simulink model "Expriment_All2"  (R2014a)
settings: Solver=FixedStepDiscrete  SolverMode=SingleTasking  StartTime=0.0  StopTime=inf  FixedStep=0.01  RelTol=1e-3
PostLoadFcn:
  | h_RPStest = RPStest;
model workspace (MAT data in the model file):
  gtest = 0
undefined symbols (not defined in the file or in its folder): avert, avert_freq_factor, avert_gaze_dirs_chance, avert_gaze_duration_factor, avert_head_frequency_factor, avert_head_speed, BML, BML1, BML2, bmlsL, bmlsM, bodyBusyFlag, clock, emotion_amount_factor, faceBusyFlag, fileID, GAZE_WIN, gazing, mut_freq_factor, mutual_gaze_duration_factor, P, pose_cat_chance, pose_chanc_factor, pose_chance_factor, pose_frequency_factor, pose_lean, pose_lean_flag, pose_speed, pose_twitch, pr, serial, STATE_BEFORE, STATE_GO, STATE_OVER, STATE_READY, Stateflow
libraries: simulink x24, instrumentlib x6, lib_affectiveChar_behavior x2, realtime_pacer_lib x2, lib_affectiveChar_input x1
(part 5 of 7)

== stateflow chart Expriment_All2/CharacterControl/idlePose_Controller ==
  note: PERSONALITY:
      | -HN: self-touching and object manipulations, non-fluencies rigid posture and minimization of random movements, erect shoulder, cross legs Lean forward tenser
      | -LN:Lean backward reclining, head lean sideway or down
      | -High arousal: self and object adaptors, body tension and random trunk
      | For more info check Burgoon and Koper, 1984.
  note: -Ekman categorized hand poses to Emblems(e.g. hand shrug for helplessness or inability ; thumbs up), illustrators, Regulators, POINTS, Adaptors (self, alter-directed), spontaneousgests, attention-based gests
      | -Picking or squeezing part of the body is aggression against the self or aggression towards others temporarily displaced onto the self;
      | -covering the eye with a hand is relevant to preventing input, avoiding being seen, and shame
      | For more infor refer to Ekman (1972) Hand Movements.
  note: continously unpdate values based on change in valence-arousal
  note: The higher BOREDOMT (treshold), the lower chance of bored pose.
  note: Logically, personality parameters should only get calculated once. Since, here we change the personality dynamically during simulation,we calculate it in each loop.
  note: Problems with priortizing behaviors:
      |     1) When personality change, we want a few adjustments to happen e.g. agent's lean pose changes. The problem is system detects the change and set the flag to 1 and then again goes back to 0. If we dont check in stateflow exactly at that time we dont detect the change. that's why we need another flag that keeps the change till we do the personality based adjustment in behavior.After doing the adjustment we set that flag to zero.
      |     2) We can not use this for tracking if the body is busy at the time. When there is environmnet change agent reacts either by face or body (faceBusyFlag and bodyBusyFlag). We want to stop sending idle BML when they are busy. We need to check if flag is 1 excatly when we want to send the idle body or gaze BML.(if its a few milisec after or before it may not be busy. That's why we need attendChange module to set the flag to 1 for 10 sec after bodyBusy or faceBusy to avoid generating idle behavior in that period.
      |     3)problem also occures when the agent is at the middle of an idle pose/avert and needs to do interactive pose. It causes averted head+smile etc.
  note: Brebner pointed out that frequency of hand movements/gestures was positively correlated with Extraversion [9].
      | Brebner, J. 1985. Personality theory and movement. In B.D. Kirkcaldy (Ed.), Individual differences in movement (pp.
      | 27-41). Lancaster, England: MTP Press Limited.
  note: Riggio suggested that extraverts change their posture more often.
      | Riggio, R., Friedman, H. 1986. Impression formation: The
      | role of expressive behavior. In Journal of Personality and
      | Social Psychology 50(2), 421-427
  state idlePoseGenerate [parallel]
    settings: executionOrder=1
    state stateInit
      entry:STATE_OVER=3;STATE_BEFORE=4;pose_lean_flag=0;
      STATE_READY=7;STATE_GO=1;gameState= 14;
      n=encStr2Arr(' ');bmlsL=[n n n n n];newBmlsL=[n n n n n];
      pose_frequency_factor=40;pose_chance_factor=1;pose_cat_chance=50;
      pose_lean=18; pose_speed=1;pose_lean_flag=0;pose_twitch=0;pose_space=0;
      poseNum=0;oldPose=0;
    state leanChange
      entry:  pose_lean_flag=0;
      [P,BMLM]=weightshift_SpaceTable(pose_lean) ;
      newBmlsM=insertQueue(bmlsM,BMLM);
      bmlsM=newBmlsM;
    state stateRandomPose
      entry: randSlowPose=randArray(:,11);%(1,4)
      interest=BOREDOM_THRESHOLD-boredom;interest=1;
    state stateExtrovertPoseChance
      entry: randPoseChance=round(randSlowPose/pose_chance_factor);
    note: SLOW
    note: FAST
    note: else
    note: else
    state poseCategoryChance1
      entry: randPR=randArray(:,20);
    state poseCategoryChance2
      entry: randPR=randArray(:,20);
    state poseCategoryChance
      entry: randPR=randArray(:,20);
    note: else
    note: else
    state selfAdaptorPoseCategory
      entry:pose_type=selfAdaptorTypeTable(pose_speed, pose_twitch);
      poseNum=randArray(:,pose_type) ;
    state weightshiftPoseCategory
      entry:pose_type=weightShiftTypeTable(pose_speed,pose_space);
      poseNum=randArray(:,pose_type);%fprintf(' space=: '); fprintf('%0.0f',pose_space);
    state avoidRepeatedPose1
      entry: poseNum=randArray(:,pose_type) ;
    state avoidRepeatedPose
      entry: poseNum=randArray(:,pose_type) ;
    state selfAdaptorPoseCategory1
      entry:oldPose=poseNum;
      [P,BMLl]=selfAdaptor_TwitchTable(poseNum);
      newBmlsL=insertQueueLow(bmlsL,BMLl);
      bmlsL=newBmlsL;%disp(decArr2Str(BMLl));
    state weightshiftPoseCategory1
      entry:
      [P,BMLl]= weightshift_SpaceTable(poseNum);
      newBmlsL=insertQueueLow(bmlsL,BMLl);
      bmlsL=newBmlsL;
    (default) -> stateInit
    stateInit -> stateRandomPose
    leanChange -> stateRandomPose : after(1,secs)
    stateRandomPose -> leanChange [order 1] : [pose_lean_flag==1]
    (junction 2) -> stateRandomPose [order 2]
    weightshiftPoseCategory1 -> stateRandomPose : after(pose_frequency_factor,secs)
    (junction 425) -> stateRandomPose [order 2]
    stateRandomPose -> stateExtrovertPoseChance [order 2]
    (junction 169) -> stateRandomPose [order 2]
    selfAdaptorPoseCategory1 -> stateRandomPose : after(pose_frequency_factor,secs)
    stateExtrovertPoseChance -> (junction 2) [order 2] : [pose_speed==2]
    stateExtrovertPoseChance -> (junction 425) [order 3] : [pose_speed==1]
    stateExtrovertPoseChance -> (junction 169) [order 1] : [pose_speed==3]
    (junction 425) -> poseCategoryChance2 [order 1] : [[randPoseChance==1]&[ gameState~= STATE_GO]&[ gameState~= STATE_READY]]
    (junction 2) -> poseCategoryChance1 [order 1] : [[randPoseChance==1]&[ gameState~= STATE_GO]&[ gameState~= STATE_READY]]
    (junction 169) -> poseCategoryChance [order 1] : [[randPoseChance==1]&[ gameState~= STATE_GO]&[ gameState~= STATE_READY]]
    poseCategoryChance2 -> poseCategoryChance2 [order 2]
    poseCategoryChance1 -> poseCategoryChance1 [order 2]
    poseCategoryChance -> poseCategoryChance [order 2]
    poseCategoryChance1 -> (junction 344) [order 1] : [bodyBusyFlag~=1]
    poseCategoryChance2 -> (junction 431) [order 1] : [bodyBusyFlag~=1]
    poseCategoryChance -> (junction 340) [order 1] : [bodyBusyFlag~=1]
    (junction 340) -> (junction 212) [order 1] : [randPR<=pose_cat_chance]
    (junction 431) -> (junction 211) [order 2] : [randPR>pose_cat_chance]
    (junction 431) -> (junction 212) [order 1] : [randPR<=pose_cat_chance]
    (junction 344) -> (junction 211) [order 1] : [randPR<=pose_cat_chance]
    (junction 340) -> (junction 211) [order 2] : [randPR>pose_cat_chance ]
    (junction 344) -> (junction 212) [order 2] : [randPR>pose_cat_chance]
    (junction 212) -> weightshiftPoseCategory
    (junction 211) -> selfAdaptorPoseCategory
    selfAdaptorPoseCategory -> avoidRepeatedPose
    weightshiftPoseCategory -> avoidRepeatedPose1
    avoidRepeatedPose1 -> avoidRepeatedPose1 [order 1] : [poseNum==oldPose]
    avoidRepeatedPose -> avoidRepeatedPose [order 1] : [poseNum==oldPose]
    avoidRepeatedPose1 -> weightshiftPoseCategory1 [order 2] : %else
    avoidRepeatedPose -> selfAdaptorPoseCategory1 [order 2] : %else
  note: randSlowPose=randi(1,6)
  note: D10 for animation 8 which is hand on waist may not work with wave etc. Too long!
  note: bml.execBML('*', '<animation name="ChrBrad@Idle01_ScratchHeadLf01" start="0" stroke="3" relax="12" end="14" />')
      | spacious poses should take long to look extrovert: continouing occupying space and being conftable with it.
      | for future work, can explore the effect of time on perception of extrovert and possibly dominant impression.
  note: McNeill's gesture space sectors: the performance space in front of an actor is divided into three gesture space sections: Center-Center (CC), Center (C), and Periphery (P). CC is the central section directly in front of the chest, while subsequent sections (C and P) form spatial layers spreading outwards. low-warmth-low-competence performance consists of gestures mostly in the lower, center P region, while high-warmth-high-competence focuses mostly in the CC and C regions.
  data: bmlID function_input double; pr function_output double size=1; poseBML function_output double size=[1000,1]; bmlID function_input double; pr function_output double size=1; poseBML function_output double size=[1000,1]; pr function_output double size=1; bmlID function_input double; poseBML function_output double size=[1000,1]; poseSpeed function_input double size=1; shiftType function_output double size=1; spacious function_input double size=1; poseSpeed function_input double size=1; poseTwitch function_input double size=1; poseType function_output double size=1; bmls function_input double size=[1000,5]; myBML function_input double size=[1000,1]; newBmls function_output double size=[1000,5]; bmls function_input double size=[1000,5]; myBML function_input double size=[1000,1]; newBmls function_output double size=[1000,5]; boredom data_store_memory size=2; BOREDOM_THRESHOLD data_store_memory size=2; randSlowPose data_store_memory size=2; interest data_store_memory size=2; gameState output double size=1; randPoseChance data_store_memory size=1; STATE_OVER data_store_memory size=2; STATE_BEFORE data_store_memory size=2; STATE_READY data_store_memory size=2; inA input double size=1; inE input double size=1; HAPPY data_store_memory size=1 =4; SAD data_store_memory size=1 =4; CONTEMPT data_store_memory size=1 =4; BORED data_store_memory size=1 =4; FRUST data_store_memory size=1 =4; FEAR data_store_memory size=1 =4; IDLE data_store_memory size=1 =4; EXCITE data_store_memory size=1 =4; BML data_store_memory size=[256,1]; P data_store_memory; fileID data_store_memory; STATE_GO data_store_memory; bodyBusyFlag data_store_memory; BMLM local double size=[1000,1]; newBmlsL local double size=[1000,5]; bmlsL data_store_memory; n local; randArray input double size=[1,40]; personality input double size=1; randPR local; pPoseChance local; poseFreq local; leanPose local; inV input double size=1; pPoseChanceP local; poseFreqP local; pCatChance local; catChance local; personalityChange input boolean size=1; bmlsM data_store_memory; BMLl local double size=[1000,1]; newBmlsM local double size=[1000,5]; pChangeFlag local; faceBusyFlag data_store_memory; poseArray input double size=[1, 6]; pose_speed data_store_memory; pose_lean_flag data_store_memory; pose_lean data_store_memory; pose_frequency_factor data_store_memory; pose_chance_factor data_store_memory; pose_cat_chance data_store_memory; pose_change_flag data_store_memory; pose_type local; pose_twitch data_store_memory; pose_space data_store_memory; poseNum local double size=1; oldPose local double size=1
  events: secs input RISING_EDGE_EVENT
  function [pr,poseBML]=selfAdaptorTableBilly(bmlID):
    | function [pr,poseBML]=selfAdaptorTableBilly(bmlID)
    | 
    | aVarTruthTableCondition_1 = false;
    | aVarTruthTableCondition_2 = false;
    | aVarTruthTableCondition_3 = false;
    | aVarTruthTableCondition_4 = false;
    | aVarTruthTableCondition_5 = false;
    | aVarTruthTableCondition_6 = false;
    | aVarTruthTableCondition_7 = false;
    | aVarTruthTableCondition_8 = false;
    | aVarTruthTableCondition_9 = false;
    | aVarTruthTableCondition_10 = false;
    | aVarTruthTableCondition_11 = false;
    | aVarTruthTableCondition_12 = false;
    | aVarTruthTableCondition_13 = false;
    | aVarTruthTableCondition_14 = false;
    | aVarTruthTableCondition_15 = false;
    | aVarTruthTableCondition_16 = false;
    | aVarTruthTableCondition_17 = false;
    | aVarTruthTableCondition_18 = false;
    | aVarTruthTableCondition_19 = false;
    | aVarTruthTableCondition_20 = false;
    | 
    | 
    | 
    | aVarTruthTableCondition_1 = logical(bmlID==1);
    | 
    | 
    | aVarTruthTableCondition_2 = logical(bmlID==2);
    | 
    | 
    | aVarTruthTableCondition_3 = logical(bmlID==3);
    | 
    | 
    | aVarTruthTableCondition_4 = logical(bmlID==4);
    | 
    | 
    | aVarTruthTableCondition_5 = logical(bmlID==5);
    | 
    | 
    | aVarTruthTableCondition_6 = logical(bmlID==6);
    | 
    | 
    | aVarTruthTableCondition_7 = logical(bmlID==7);
    | 
    | 
    | aVarTruthTableCondition_8 = logical(bmlID==8);
    | 
    | 
    | aVarTruthTableCondition_9 = logical(bmlID==9);
    | 
    | 
    | aVarTruthTableCondition_10 = logical(bmlID==10);
    | 
    | 
    | aVarTruthTableCondition_11 = logical(bmlID==11);
    | 
    | 
    | aVarTruthTableCondition_12 = logical(bmlID==12);
    | 
    | 
    | aVarTruthTableCondition_13 = logical(bmlID==13);
    | 
    | 
    | aVarTruthTableCondition_14 = logical(bmlID==14);
    | 
    | 
    | aVarTruthTableCondition_15 = logical(bmlID==15);
    | 
    | 
    | aVarTruthTableCondition_16 = logical(bmlID==16);
    | 
    | 
    | aVarTruthTableCondition_17 = logical(bmlID==17);
    | 
    | 
    | aVarTruthTableCondition_18 = logical(bmlID==18);
    | 
    | 
    | aVarTruthTableCondition_19 = logical(bmlID==19);
    | 
    | 
    | aVarTruthTableCondition_20 = logical(bmlID==20);
    | 
    | if (aVarTruthTableCondition_1)
    |     aFcnTruthTableAction_1();
    | elseif (aVarTruthTableCondition_2)
    |     aFcnTruthTableAction_2();
    | elseif (aVarTruthTableCondition_3)
    |     aFcnTruthTableAction_3();
    | elseif (aVarTruthTableCondition_4)
    |     aFcnTruthTableAction_4();
    | elseif (aVarTruthTableCondition_5)
    |     aFcnTruthTableAction_5();
    | elseif (aVarTruthTableCondition_6)
    |     aFcnTruthTableAction_6();
    | elseif (aVarTruthTableCondition_7)
    |     aFcnTruthTableAction_7();
    | elseif (aVarTruthTableCondition_8)
    |     aFcnTruthTableAction_8();
    | elseif (aVarTruthTableCondition_9)
    |     aFcnTruthTableAction_9();
    | elseif (aVarTruthTableCondition_10)
    |     aFcnTruthTableAction_10();
    | elseif (aVarTruthTableCondition_11)
    |     aFcnTruthTableAction_11();
    | elseif (aVarTruthTableCondition_12)
    |     aFcnTruthTableAction_12();
    | elseif (aVarTruthTableCondition_13)
    |     aFcnTruthTableAction_13();
    | elseif (aVarTruthTableCondition_14)
    |     aFcnTruthTableAction_14();
    | elseif (aVarTruthTableCondition_15)
    |     aFcnTruthTableAction_15();
    | elseif (aVarTruthTableCondition_16)
    |     aFcnTruthTableAction_16();
    | elseif (aVarTruthTableCondition_17)
    |     aFcnTruthTableAction_17();
    | elseif (aVarTruthTableCondition_18)
    |     aFcnTruthTableAction_18();
    | elseif (aVarTruthTableCondition_19)
    |     aFcnTruthTableAction_19();
    | elseif (aVarTruthTableCondition_20)
    |     aFcnTruthTableAction_20();
    | else % Default
    |     aFcnTruthTableAction_1();
    | end
    | 
    | function aFcnTruthTableAction_1()
    | 
    | % WeightShiftFast
    | 
    | poseBML=encStr2Arr('<?xml version="1.0" ?><act><bml><animation name="ChrBrad@Idle01_WeightShift01" speed="2" /></bml></act>');pr=3;
    | 
    | function aFcnTruthTableAction_2()
    | 
    | % WeightShift2F
    | 
    | poseBML=encStr2Arr('<?xml version="1.0" ?><act><bml><animation name="ChrBrad@Idle01_WeightShift02" speed="2"/></bml></act>'); pr=3;
    | 
    | function aFcnTruthTableAction_3()
    | 
    | % ShoulderStretchUpDownF
    | 
    | poseBML=encStr2Arr('<?xml version="1.0" ?><act><bml><animation name="ChrBrad@Idle01_ShoulderStretch01" speed="2"/></bml></act>');pr=3;
    | 
    | function aFcnTruthTableAction_4()
    | 
    | % ScratchHeadF
    | 
    | poseBML=encStr2Arr('<?xml version="1.0" ?><act><bml><animation name="ChrBrad@Idle01_ScratchHeadLf01" speed="2"/></bml></act>'); pr=3;
    | 
    | function aFcnTruthTableAction_5()
    | 
    | % scratchtemple(head)F
    | 
    | poseBML=encStr2Arr('<?xml version="1.0" ?><act><bml><animation name="ChrBrad@Idle01_ScratchTempleLf01" speed="2"/></bml></act>'); pr=3;
    | 
    | function aFcnTruthTableAction_6()
    | 
    | % ScratchChestF
    | 
    | poseBML=encStr2Arr('<?xml version="1.0" ?><act><bml><animation name="ChrBrad@Idle01_ScratchChest01" speed="2"/></bml></act>');pr=3;
    | 
    | function aFcnTruthTableAction_7()
    | 
    | % SqueezeHand01F
    | 
    | poseBML=encStr2Arr('<?xml version="1.0" ?><act><bml><animation name="ChrBrad@Idle01_SqueezeHand01" speed="2" /></bml></act>');pr=3;
    | 
    | function aFcnTruthTableAction_8()
    | 
    | % brushCenterF
    | 
    | poseBML=encStr2Arr('<?xml version="1.0" ?><act><bml><gaze angle="10" direction="DOWNLEFT" sbm:joint-range="EYES NECK" sbm:time-hint="2" target="gazeTarget"/><gaze angle="20" direction="DOWNLEFT" sbm:joint-range="EYES" sbm:time-hint="2" target="gazeTarget"/><animation name="../data/ChrBrad/test_idle_brush_center.skm" speed="2"/></bml></act>'); pr=3;
    | 
    | function aFcnTruthTableAction_9()
    | 
    | % lookHandF
    | 
    | poseBML=encStr2Arr('<?xml version="1.0" ?><act><bml><gaze angle="10" direction="DOWNRIGHT" sbm:joint-range="EYES NECK" sbm:time-hint="2" target="gazeTarget"/><gaze angle="20" direction="DOWNRIGHT" sbm:joint-range="EYES" sbm:time-hint="2" target="gazeTarget"/><animation name="../data/ChrBrad/test_idle_hand_look.skm" speed="2"/></bml></act>'); pr=3;
    | 
    | function aFcnTruthTableAction_10()
    | 
    | % TouchHands01Slow-introvert
    | 
    | poseBML=encStr2Arr('<?xml version="1.0" ?><act><bml><animation name="ChrBrad@Idle01_TouchHands01" speed="0.8" /></bml></act>');pr=3;
    | 
    | function aFcnTruthTableAction_11()
    | 
    | % ScratchChestSlow
    | 
    | poseBML=encStr2Arr('<?xml version="1.0" ?><act><bml><animation name="ChrBrad@Idle01_ScratchChest01" speed="1"/></bml></act>');pr=3;
    | 
    | function aFcnTruthTableAction_12()
    | 
    | % WeightShiftSlow
    | 
    | poseBML=encStr2Arr('<?xml version="1.0" ?><act><bml><animation name="ChrBrad@Idle01_WeightShift01" speed="1" /></bml></act>');pr=3;
    | 
    | function aFcnTruthTableAction_13()
    | 
    | % scratchtempleSlow
    | 
    | poseBML=encStr2Arr('<?xml version="1.0" ?><act><bml><animation name="ChrBrad@Idle01_ScratchTempleLf01" speed="1" /></bml></act>');pr=3;
    | 
    | function aFcnTruthTableAction_14()
    | 
    | % SqueezeHandSlow
    | 
    | poseBML=encStr2Arr('<?xml version="1.0" ?><act><bml><animation name="ChrBrad@Idle01_SqueezeHand01" speed="1" /></bml></act>');pr=3;
    | 
    | function aFcnTruthTableAction_15()
    | 
    | % SqueezeHandSlowest
    | 
    | poseBML=encStr2Arr('<?xml version="1.0" ?><act><bml><animation name="ChrBrad@Idle01_SqueezeHand01" speed="0.7" /></bml></act>');pr=3;
    | 
    | function aFcnTruthTableAction_16()
    | 
    | % ShoulderStretchUpDownSlow
    | 
    | poseBML=encStr2Arr('<?xml version="1.0" ?><act><bml><animation name="ChrBrad@Idle01_ShoulderStretch01" speed="1"/></bml></act>');pr=3;
    | 
    | function aFcnTruthTableAction_17()
    | 
    | % WeightShift2Slow
    | 
    | poseBML=encStr2Arr('<?xml version="1.0" ?><act><bml><animation name="ChrBrad@Idle01_WeightShift02" speed="1"/></bml></act>'); pr=3;
    | 
    | function aFcnTruthTableAction_18()
    | 
    | % brushArmS
    | 
    | poseBML=encStr2Arr('<?xml version="1.0" ?><act><bml><gaze angle="20" direction="DOWNLEFT" sbm:joint-range="EYES NECK" sbm:time-hint="1" target="gazeTarget"/><gaze angle="30" direction="DOWNLEFT" sbm:joint-range="EYES" sbm:time-hint="1" target="gazeTarget"/><animation name="../data/ChrBrad/test_idle_brush.skm" speed="1"/></bml></act>'); pr=3;
    | 
    | function aFcnTruthTableAction_19()
    | 
    | % brushChestS
    | 
    | poseBML=encStr2Arr('<?xml version="1.0" ?><act><bml><gaze angle="10" direction="DOWNLEFT" sbm:joint-range="EYES NECK" sbm:time-hint="1" target="gazeTarget"/><gaze angle="20" direction="DOWNLEFT" sbm:joint-range="EYES" sbm:time-hint="1" target="gazeTarget"/><animation name="../data/ChrBrad/test_idle_brush_center.skm" speed="1"/></bml></act>'); pr=3;
    | 
    | function aFcnTruthTableAction_20()
    | 
    | % gazeAtHandS
    | 
    | poseBML=encStr2Arr('<?xml version="1.0" ?><act><bml><gaze angle="10" direction="DOWNRIGHT" sbm:joint-range="EYES NECK" sbm:time-hint="1" target="gazeTarget"/><gaze angle="20" direction="DOWNRIGHT" sbm:joint-range="EYES" sbm:time-hint="1" target="gazeTarget"/><animation name="../data/ChrBrad/test_idle_hand_look.skm" speed="1"/></bml></act>'); pr=3;
  function [pr,poseBML]=selfAdaptor_TwitchTable(bmlID):
    | function [pr,poseBML]=selfAdaptor_TwitchTable(bmlID)
    | 
    | aVarTruthTableCondition_1 = false;
    | aVarTruthTableCondition_2 = false;
    | aVarTruthTableCondition_3 = false;
    | aVarTruthTableCondition_4 = false;
    | aVarTruthTableCondition_5 = false;
    | aVarTruthTableCondition_6 = false;
    | aVarTruthTableCondition_7 = false;
    | aVarTruthTableCondition_8 = false;
    | aVarTruthTableCondition_9 = false;
    | aVarTruthTableCondition_10 = false;
    | aVarTruthTableCondition_11 = false;
    | aVarTruthTableCondition_12 = false;
    | aVarTruthTableCondition_13 = false;
    | aVarTruthTableCondition_14 = false;
    | aVarTruthTableCondition_15 = false;
    | aVarTruthTableCondition_16 = false;
    | aVarTruthTableCondition_17 = false;
    | aVarTruthTableCondition_18 = false;
    | aVarTruthTableCondition_19 = false;
    | aVarTruthTableCondition_20 = false;
    | aVarTruthTableCondition_21 = false;
    | aVarTruthTableCondition_22 = false;
    | aVarTruthTableCondition_23 = false;
    | aVarTruthTableCondition_24 = false;
    | aVarTruthTableCondition_25 = false;
    | 
    | 
    | 
    | aVarTruthTableCondition_1 = logical(bmlID==1);
    | 
    | 
    | aVarTruthTableCondition_2 = logical(bmlID==2);
    | 
    | 
    | aVarTruthTableCondition_3 = logical(bmlID==3);
    | 
    | 
    | aVarTruthTableCondition_4 = logical(bmlID==4);
    | 
    | 
    | aVarTruthTableCondition_5 = logical(bmlID==5);
    | 
    | 
    | aVarTruthTableCondition_6 = logical(bmlID==6);
    | 
    | 
    | aVarTruthTableCondition_7 = logical(bmlID==7);
    | 
    | 
    | aVarTruthTableCondition_8 = logical(bmlID==8);
    | 
    | 
    | aVarTruthTableCondition_9 = logical(bmlID==9);
    | 
    | 
    | aVarTruthTableCondition_10 = logical(bmlID==10);
    | 
    | 
    | aVarTruthTableCondition_11 = logical(bmlID==11);
    | 
    | 
    | aVarTruthTableCondition_12 = logical(bmlID==12);
    | 
    | 
    | aVarTruthTableCondition_13 = logical(bmlID==13);
    | 
    | 
    | aVarTruthTableCondition_14 = logical(bmlID==14);
    | 
    | 
    | aVarTruthTableCondition_15 = logical(bmlID==15);
    | 
    | 
    | aVarTruthTableCondition_16 = logical(bmlID==16);
    | 
    | 
    | aVarTruthTableCondition_17 = logical(bmlID==17);
    | 
    | 
    | aVarTruthTableCondition_18 = logical(bmlID==18);
    | 
    | 
    | aVarTruthTableCondition_19 = logical(bmlID==19);
    | 
    | 
    | aVarTruthTableCondition_20 = logical(bmlID==20);
    | 
    | 
    | aVarTruthTableCondition_21 = logical(bmlID==21);
    | 
    | 
    | aVarTruthTableCondition_22 = logical(bmlID==22);
    | 
    | 
    | aVarTruthTableCondition_23 = logical(bmlID==23);
    | 
    | 
    | aVarTruthTableCondition_24 = logical(bmlID==24);
    | 
    | 
    | aVarTruthTableCondition_25 = logical(bmlID==25);
    | 
    | if (aVarTruthTableCondition_1)
    |     aFcnTruthTableAction_1();
    | elseif (aVarTruthTableCondition_2)
    |     aFcnTruthTableAction_2();
    | elseif (aVarTruthTableCondition_3)
    |     aFcnTruthTableAction_3();
    | elseif (aVarTruthTableCondition_4)
    |     aFcnTruthTableAction_4();
    | elseif (aVarTruthTableCondition_5)
    |     aFcnTruthTableAction_5();
    | elseif (aVarTruthTableCondition_6)
    |     aFcnTruthTableAction_6();
    | elseif (aVarTruthTableCondition_7)
    |     aFcnTruthTableAction_7();
    | elseif (aVarTruthTableCondition_8)
    |     aFcnTruthTableAction_8();
    | elseif (aVarTruthTableCondition_9)
    |     aFcnTruthTableAction_9();
    | elseif (aVarTruthTableCondition_10)
    |     aFcnTruthTableAction_10();
    | elseif (aVarTruthTableCondition_11)
    |     aFcnTruthTableAction_11();
    | elseif (aVarTruthTableCondition_12)
    |     aFcnTruthTableAction_12();
    | elseif (aVarTruthTableCondition_13)
    |     aFcnTruthTableAction_13();
    | elseif (aVarTruthTableCondition_14)
    |     aFcnTruthTableAction_14();
    | elseif (aVarTruthTableCondition_15)
    |     aFcnTruthTableAction_15();
    | elseif (aVarTruthTableCondition_16)
    |     aFcnTruthTableAction_16();
    | elseif (aVarTruthTableCondition_17)
    |     aFcnTruthTableAction_17();
    | elseif (aVarTruthTableCondition_18)
    |     aFcnTruthTableAction_18();
    | elseif (aVarTruthTableCondition_19)
    |     aFcnTruthTableAction_19();
    | elseif (aVarTruthTableCondition_20)
    |     aFcnTruthTableAction_20();
    | elseif (aVarTruthTableCondition_21)
    |     aFcnTruthTableAction_21();
    | elseif (aVarTruthTableCondition_22)
    |     aFcnTruthTableAction_22();
    | elseif (aVarTruthTableCondition_23)
    |     aFcnTruthTableAction_23();
    | elseif (aVarTruthTableCondition_24)
    |     aFcnTruthTableAction_24();
    | elseif (aVarTruthTableCondition_25)
    |     aFcnTruthTableAction_25();
    | else % Default
    |     aFcnTruthTableAction_1();
    | end
    | 
    | function aFcnTruthTableAction_1()
    | 
    | % ScratchHeadNormal
    | 
    | poseBML=encStr2Arr('<?xml version="1.0" ?><act><bml><animation name="ChrBrad@Idle01_ScratchHeadLf01" speed="1"/></bml></act>'); pr=3;
    | 
    | function aFcnTruthTableAction_2()
    | 
    | % scratchtemple(head)Normal
    | 
    | poseBML=encStr2Arr('<?xml version="1.0" ?><act><bml><animation name="ChrBrad@Idle01_ScratchTempleLf01" speed="1"/></bml></act>'); pr=3;
    | 
    | function aFcnTruthTableAction_3()
    | 
    | % ScratchChestNormal
    | 
    | poseBML=encStr2Arr('<?xml version="1.0" ?><act><bml><animation name="ChrBrad@Idle01_ScratchChest01" speed="1"/></bml></act>');pr=3;
    | 
    | function aFcnTruthTableAction_4()
    | 
    | % TouchHands01Norm
    | 
    | poseBML=encStr2Arr('<?xml version="1.0" ?><act><bml><animation name="ChrBrad@Idle01_TouchHands01" speed="1" /></bml></act>');pr=3;
    | 
    | function aFcnTruthTableAction_5()
    | 
    | % SqueezeHand01Norm
    | 
    | poseBML=encStr2Arr('<?xml version="1.0" ?><act><bml><animation name="ChrBrad@Idle01_SqueezeHand01"  speed="1"/></bml></act>');pr=3;
    | 
    | function aFcnTruthTableAction_6()
    | 
    | % TouchHands01F
    | 
    | poseBML=encStr2Arr('<?xml version="1.0" ?><act><bml><animation name="ChrBrad@Idle01_TouchHands01" speed="1.5" /></bml></act>');pr=3;
    | 
    | function aFcnTruthTableAction_7()
    | 
    | % TouchHands01F2
    | 
    | poseBML=encStr2Arr('<?xml version="1.0" ?><act><bml><animation name="ChrBrad@Idle01_TouchHands01" speed="1.3" /></bml></act>');pr=3;
    | 
    | function aFcnTruthTableAction_8()
    | 
    | % squeezeHandF3
    | 
    | poseBML=encStr2Arr('<?xml version="1.0" ?><act><bml><animation name="ChrBrad@Idle01_SqueezeHand01" speed="1.7" /></bml></act>');pr=3;
    | 
    | function aFcnTruthTableAction_9()
    | 
    | % ScratchChestF
    | 
    | poseBML=encStr2Arr('<?xml version="1.0" ?><act><bml><animation name="ChrBrad@Idle01_ScratchChest01" speed="1.5"/></bml></act>');pr=3;
    | 
    | function aFcnTruthTableAction_10()
    | 
    | % scratchtempleF
    | 
    | poseBML=encStr2Arr('<?xml version="1.0" ?><act><bml><animation name="ChrBrad@Idle01_ScratchTempleLf01" speed="1.5" /></bml></act>');pr=3;
    | 
    | function aFcnTruthTableAction_11()
    | 
    | % scratchHeadF2
    | 
    | poseBML=encStr2Arr('<?xml version="1.0" ?><act><bml><animation name="ChrBrad@Idle01_ScratchHeadLf01" speed="1.6"/></bml></act>');pr=3;
    | 
    | function aFcnTruthTableAction_12()
    | 
    | % SqueezeHandF1
    | 
    | poseBML=encStr2Arr('<?xml version="1.0" ?><act><bml><animation name="ChrBrad@Idle01_SqueezeHand01" speed="1.5" /></bml></act>');pr=3;
    | 
    | function aFcnTruthTableAction_13()
    | 
    | % SqueezeHandF2
    | 
    | poseBML=encStr2Arr('<?xml version="1.0" ?><act><bml><animation name="ChrBrad@Idle01_SqueezeHand01" speed="1.2" /></bml></act>');pr=3;
    | 
    | function aFcnTruthTableAction_14()
    | 
    | % ScratchHeadF
    | 
    | poseBML=encStr2Arr('<?xml version="1.0" ?><act><bml><animation name="ChrBrad@Idle01_ScratchHeadLf01" speed="1.5"/></bml></act>'); pr=3;
    | 
    | function aFcnTruthTableAction_15()
    | 
    | % twitchFast
    | 
    | poseBML=encStr2Arr('<?xml version="1.0" ?><act><bml><animation name="ChrBrad@Idle01_ShoulderStretch01" speed="3"/></bml></act>');pr=3;
    | 
    | function aFcnTruthTableAction_16()
    | 
    | % SqueezeHandS2
    | 
    | poseBML=encStr2Arr('<?xml version="1.0" ?><act><bml><animation name="ChrBrad@Idle01_SqueezeHand01" speed="0.5" /></bml></act>');pr=3;
    | 
    | function aFcnTruthTableAction_17()
    | 
    | % ScratchHeadS
    | 
    | poseBML=encStr2Arr('<?xml version="1.0" ?><act><bml><animation name="ChrBrad@Idle01_ScratchHeadLf01" speed="0.6"/></bml></act>'); pr=3;
    | 
    | function aFcnTruthTableAction_18()
    | 
    | % scratchtemple(head)S
    | 
    | poseBML=encStr2Arr('<?xml version="1.0" ?><act><bml><animation name="ChrBrad@Idle01_ScratchTempleLf01" speed="0.6"/></bml></act>'); pr=3;
    | 
    | function aFcnTruthTableAction_19()
    | 
    | % ScratchChestS
    | 
    | poseBML=encStr2Arr('<?xml version="1.0" ?><act><bml><animation name="ChrBrad@Idle01_ScratchChest01" speed="0.6"/></bml></act>');pr=3;
    | 
    | function aFcnTruthTableAction_20()
    | 
    | % TouchHands01S
    | 
    | poseBML=encStr2Arr('<?xml version="1.0" ?><act><bml><animation name="ChrBrad@Idle01_TouchHands01" speed="0.8" /></bml></act>');pr=3;
    | 
    | function aFcnTruthTableAction_21()
    | 
    | % TouchHands01S2
    | 
    | poseBML=encStr2Arr('<?xml version="1.0" ?><act><bml><animation name="ChrBrad@Idle01_TouchHands01" speed="0.9" /></bml></act>');pr=3;
    | 
    | function aFcnTruthTableAction_22()
    | 
    | % squeezeHand S3
    | 
    | poseBML=encStr2Arr('<?xml version="1.0" ?><act><bml><animation name="ChrBrad@Idle01_SqueezeHand01" speed="0.7" /></bml></act>');pr=3;
    | 
    | function aFcnTruthTableAction_23()
    | 
    | % head slow2
    | 
    | poseBML=encStr2Arr('<?xml version="1.0" ?><act><bml><animation name="ChrBrad@Idle01_ScratchHeadLf01" speed="0.7"/></bml></act>');pr=3;
    | 
    | function aFcnTruthTableAction_24()
    | 
    | % SqueezeHand01S
    | 
    | poseBML=encStr2Arr('<?xml version="1.0" ?><act><bml><animation name="ChrBrad@Idle01_SqueezeHand01"  speed="0.6"/></bml></act>');pr=3;
    | 
    | function aFcnTruthTableAction_25()
    | 
    | % twitchS
    | 
    | poseBML=encStr2Arr('<?xml version="1.0" ?><act><bml><animation name="ChrBrad@Idle01_ShoulderStretch01" speed="2"/></bml></act>');pr=3;
  function [pr,poseBML]=weightshift_SpaceTable(bmlID):
    | function [pr,poseBML]=weightshift_SpaceTable(bmlID)
    | 
    | aVarTruthTableCondition_1 = false;
    | aVarTruthTableCondition_2 = false;
    | aVarTruthTableCondition_3 = false;
    | aVarTruthTableCondition_4 = false;
    | aVarTruthTableCondition_5 = false;
    | aVarTruthTableCondition_6 = false;
    | aVarTruthTableCondition_7 = false;
    | aVarTruthTableCondition_8 = false;
    | aVarTruthTableCondition_9 = false;
    | aVarTruthTableCondition_10 = false;
    | aVarTruthTableCondition_11 = false;
    | aVarTruthTableCondition_12 = false;
    | aVarTruthTableCondition_13 = false;
    | aVarTruthTableCondition_14 = false;
    | aVarTruthTableCondition_15 = false;
    | aVarTruthTableCondition_16 = false;
    | aVarTruthTableCondition_17 = false;
    | aVarTruthTableCondition_18 = false;
    | aVarTruthTableCondition_19 = false;
    | 
    | 
    | 
    | aVarTruthTableCondition_1 = logical(bmlID==1);
    | 
    | 
    | aVarTruthTableCondition_2 = logical(bmlID==2);
    | 
    | 
    | aVarTruthTableCondition_3 = logical(bmlID==3);
    | 
    | 
    | aVarTruthTableCondition_4 = logical(bmlID==4);
    | 
    | 
    | aVarTruthTableCondition_5 = logical(bmlID==5);
    | 
    | 
    | aVarTruthTableCondition_6 = logical(bmlID==6);
    | 
    | 
    | aVarTruthTableCondition_7 = logical(bmlID==7);
    | 
    | 
    | aVarTruthTableCondition_8 = logical(bmlID==8);
    | 
    | 
    | aVarTruthTableCondition_9 = logical(bmlID==9);
    | 
    | 
    | aVarTruthTableCondition_10 = logical(bmlID==10);
    | 
    | 
    | aVarTruthTableCondition_11 = logical(bmlID==11);
    | 
    | 
    | aVarTruthTableCondition_12 = logical(bmlID==12);
    | 
    | 
    | aVarTruthTableCondition_13 = logical(bmlID==13);
    | 
    | 
    | aVarTruthTableCondition_14 = logical(bmlID==14);
    | 
    | 
    | aVarTruthTableCondition_15 = logical(bmlID==15);
    | 
    | 
    | aVarTruthTableCondition_16 = logical(bmlID==16);
    | 
    | 
    | aVarTruthTableCondition_17 = logical(bmlID==17);
    | 
    | 
    | aVarTruthTableCondition_18 = logical(bmlID==18);
    | 
    | 
    | aVarTruthTableCondition_19 = logical(bmlID==19);
    | 
    | if (aVarTruthTableCondition_1)
    |     aFcnTruthTableAction_1();
    | elseif (aVarTruthTableCondition_2)
    |     aFcnTruthTableAction_2();
    | elseif (aVarTruthTableCondition_3)
    |     aFcnTruthTableAction_3();
    | elseif (aVarTruthTableCondition_4)
    |     aFcnTruthTableAction_4();
    | elseif (aVarTruthTableCondition_5)
    |     aFcnTruthTableAction_5();
    | elseif (aVarTruthTableCondition_6)
    |     aFcnTruthTableAction_6();
    | elseif (aVarTruthTableCondition_7)
    |     aFcnTruthTableAction_7();
    | elseif (aVarTruthTableCondition_8)
    |     aFcnTruthTableAction_8();
    | elseif (aVarTruthTableCondition_9)
    |     aFcnTruthTableAction_9();
    | elseif (aVarTruthTableCondition_10)
    |     aFcnTruthTableAction_10();
    | elseif (aVarTruthTableCondition_11)
    |     aFcnTruthTableAction_11();
    | elseif (aVarTruthTableCondition_12)
    |     aFcnTruthTableAction_12();
    | elseif (aVarTruthTableCondition_13)
    |     aFcnTruthTableAction_13();
    | elseif (aVarTruthTableCondition_14)
    |     aFcnTruthTableAction_14();
    | elseif (aVarTruthTableCondition_15)
    |     aFcnTruthTableAction_15();
    | elseif (aVarTruthTableCondition_16)
    |     aFcnTruthTableAction_16();
    | elseif (aVarTruthTableCondition_17)
    |     aFcnTruthTableAction_17();
    | elseif (aVarTruthTableCondition_18)
    |     aFcnTruthTableAction_18();
    | elseif (aVarTruthTableCondition_19)
    |     aFcnTruthTableAction_19();
    | else % Default
    |     aFcnTruthTableAction_1();
    | end
    | 
    | function aFcnTruthTableAction_1()
    | 
    | % brushCenterFast-space
    | 
    | poseBML=encStr2Arr('<?xml version="1.0" ?><act><bml><animation name="../data/ChrBrad/test_idle_brush_center.skm" speed="1.5"/></bml></act>'); pr=3;
    | 
    | function aFcnTruthTableAction_2()
    | 
    | % look hand fast-space
    | 
    | poseBML=encStr2Arr('<?xml version="1.0" ?><act><bml><gaze angle="10" direction="DOWNRIGHT" sbm:joint-range="EYES NECK" sbm:time-hint="2" target="gazeTarget"/><gaze angle="20" direction="DOWNRIGHT" sbm:joint-range="EYES" sbm:time-hint="2" target="gazeTarget"/><animation name="../data/ChrBrad/test_idle_hand_look.skm" speed="1.5"/></bml></act>'); pr=3;
    | 
    | function aFcnTruthTableAction_3()
    | 
    | % hands on waist Fast-space
    | 
    | poseBML=encStr2Arr('<?xml version="1.0" ?><act><bml><animation name="ChrBrad@Idle01_ToIdle03" start="0" ready="1" stroke="2" stroke_end="3" relax="18" end="20"/></bml></act>');pr=4;
    | 
    | function aFcnTruthTableAction_4()
    | 
    | % one hand waist Fast-space
    | 
    | poseBML=encStr2Arr('<?xml version="1.0" ?><act><bml><animation name="ChrBrad@Idle01_Think01" start="0" ready="1" stroke="4" stroke_end="20"  relax="21" end="22" /></bml></act>');pr=4;
    | 
    | function aFcnTruthTableAction_5()
    | 
    | % armStretchFWFast-space
    | 
    | poseBML=encStr2Arr('<?xml version="1.0" ?><act><bml><animation name="ChrBrad@Idle01_ArmStretch01" speed="1.5"/></bml></act>');pr=4;
    | 
    | function aFcnTruthTableAction_6()
    | 
    | % wieghtShiftFast
    | 
    | poseBML=encStr2Arr('<?xml version="1.0" ?><act><bml><animation name="ChrBrad@Idle01_ToIdle02" speed="1.4"/></bml></act>');pr=3;
    | 
    | function aFcnTruthTableAction_7()
    | 
    | % wieghtShiftFast2
    | 
    | poseBML=encStr2Arr('<?xml version="1.0" ?><act><bml><animation name="ChrBrad@Idle01_ToIdle02" speed="1.5"/></bml></act>');pr=3;
    | 
    | function aFcnTruthTableAction_8()
    | 
    | % wieghtShiftFast3
    | 
    | poseBML=encStr2Arr('<?xml version="1.0" ?><act><bml><animation name="ChrBrad@Idle01_ToIdle02" speed="1.6"/></bml></act>');pr=3;
    | 
    | function aFcnTruthTableAction_9()
    | 
    | % ShoulderStretchUpDownFast
    | 
    | poseBML=encStr2Arr('<?xml version="1.0" ?><act><bml><animation name="ChrBrad@Idle01_ShoulderStretch01" speed="0.3"/></bml></act>');pr=3;
    | 
    | function aFcnTruthTableAction_10()
    | 
    | % ShoulderStretchUpDownNormal
    | 
    | poseBML=encStr2Arr('<?xml version="1.0" ?><act><bml><animation name="ChrBrad@Idle01_ShoulderStretch01" speed="0.2"/></bml></act>');pr=3;
    | 
    | function aFcnTruthTableAction_11()
    | 
    | % Idle01_ToIdle02Normal
    | 
    | poseBML=encStr2Arr('<?xml version="1.0" ?><act><bml><animation name="ChrBrad@Idle01_ToIdle02" speed="0.8"/></bml></act>');pr=4;
    | 
    | function aFcnTruthTableAction_12()
    | 
    | % Idle01_ToIdle02Normal2
    | 
    | poseBML=encStr2Arr('<?xml version="1.0" ?><act><bml><animation name="ChrBrad@Idle01_ToIdle02" speed="0.9"/></bml></act>');pr=4;
    | 
    | function aFcnTruthTableAction_13()
    | 
    | % Idle01_ToIdle02Normal3
    | 
    | poseBML=encStr2Arr('<?xml version="1.0" ?><act><bml><animation name="ChrBrad@Idle01_ToIdle02" speed="1"/></bml></act>');pr=4;
    | 
    | function aFcnTruthTableAction_14()
    | 
    | % Idle01_ToIdle02Slow1
    | 
    | poseBML=encStr2Arr('<?xml version="1.0" ?><act><bml><animation name="ChrBrad@Idle01_ToIdle02" speed="0.5"/></bml></act>');pr=4;
    | 
    | function aFcnTruthTableAction_15()
    | 
    | % Idle01_ToIdle02Slow2
    | 
    | poseBML=encStr2Arr('<?xml version="1.0" ?><act><bml><animation name="ChrBrad@Idle01_ToIdle02" speed="0.6"/></bml></act>');pr=4;
    | 
    | function aFcnTruthTableAction_16()
    | 
    | % Idle01_ToIdle02Slow3
    | 
    | poseBML=encStr2Arr('<?xml version="1.0" ?><act><bml><animation name="ChrBrad@Idle01_ToIdle02" speed="0.7"/></bml></act>');pr=4;
    | 
    | function aFcnTruthTableAction_17()
    | 
    | % ShoulderStretchUpDownSlow
    | 
    | poseBML=encStr2Arr('<?xml version="1.0" ?><act><bml><animation name="ChrBrad@Idle01_ShoulderStretch01" speed="0.1"/></bml></act>');pr=3;
    | 
    | function aFcnTruthTableAction_18()
    | 
    | % LeanBack-extrovert
    | 
    | poseBML=encStr2Arr('<?xml version="1.0" ?><act><bml><gaze angle="3" direction="UP" sbm:joint-range="HEAD CHEST" sbm:time-hint="2" target="gazeTarget"/></bml></act>'); pr=3;
    | 
    | function aFcnTruthTableAction_19()
    | 
    | % LeanFW-introvert
    | 
    | poseBML=encStr2Arr('<?xml version="1.0" ?><act><bml><gaze angle="3" direction="DOWN" sbm:joint-range="HEAD CHEST" sbm:time-hint="2" target="gazeTarget"/></bml></act>'); pr=3;
  function shiftType = weightShiftTypeTable(poseSpeed, spacious):
    | function shiftType = weightShiftTypeTable(poseSpeed, spacious)
    | 
    | aVarTruthTableCondition_1 = false;
    | aVarTruthTableCondition_2 = false;
    | aVarTruthTableCondition_3 = false;
    | aVarTruthTableCondition_4 = false;
    | 
    | 
    | % Fast-NoSpace
    | 
    | aVarTruthTableCondition_1 = logical([[poseSpeed==2]&&[spacious==0]]);
    | 
    | % fast-space
    | 
    | aVarTruthTableCondition_2 = logical([[poseSpeed==2]&&[spacious==1]]);
    | 
    | % Slow
    | 
    | aVarTruthTableCondition_3 = logical([poseSpeed==3]);
    | 
    | % Normal
    | 
    | aVarTruthTableCondition_4 = logical([poseSpeed==1]);
    | 
    | if (aVarTruthTableCondition_1)
    |     aFcnTruthTableAction_1();
    | elseif (aVarTruthTableCondition_2)
    |     aFcnTruthTableAction_2();
    | elseif (aVarTruthTableCondition_3)
    |     aFcnTruthTableAction_3();
    | elseif (aVarTruthTableCondition_4)
    |     aFcnTruthTableAction_4();
    | else % Default
    |     aFcnTruthTableAction_4();
    | end
    | 
    | function aFcnTruthTableAction_1()
    | 
    | % FastNoSpace
    | 
    | shiftType=21;
    | 
    | function aFcnTruthTableAction_2()
    | 
    | % fastSpace
    | 
    | shiftType=26;
    | 
    | function aFcnTruthTableAction_3()
    | 
    | % SlowWS
    | 
    | shiftType=22;
    | 
    | function aFcnTruthTableAction_4()
    | 
    | % normalWS
    | 
    | shiftType=16;
  function poseType = selfAdaptorTypeTable(poseSpeed, poseTwitch):
    | function poseType = selfAdaptorTypeTable(poseSpeed, poseTwitch)
    | 
    | aVarTruthTableCondition_1 = false;
    | aVarTruthTableCondition_2 = false;
    | aVarTruthTableCondition_3 = false;
    | aVarTruthTableCondition_4 = false;
    | aVarTruthTableCondition_5 = false;
    | 
    | 
    | % Fast-Twitch
    | 
    | aVarTruthTableCondition_1 = logical([[poseSpeed==2]&[poseTwitch==1]]);
    | 
    | % Slow-Twitch
    | 
    | aVarTruthTableCondition_2 = logical([[poseSpeed==3]&[poseTwitch==1]]);
    | 
    | % Fast-NoTwitch
    | 
    | aVarTruthTableCondition_3 = logical([[poseSpeed==2]&[poseTwitch==0]]);
    | 
    | % Slow-NoTwitch
    | 
    | aVarTruthTableCondition_4 = logical([[poseSpeed==3]&[poseTwitch==0]]);
    | 
    | % normal
    | 
    | aVarTruthTableCondition_5 = logical([poseSpeed==1]);
    | 
    | if (aVarTruthTableCondition_1)
    |     aFcnTruthTableAction_1();
    | elseif (aVarTruthTableCondition_2)
    |     aFcnTruthTableAction_2();
    | elseif (aVarTruthTableCondition_3)
    |     aFcnTruthTableAction_3();
    | elseif (aVarTruthTableCondition_4)
    |     aFcnTruthTableAction_4();
    | elseif (aVarTruthTableCondition_5)
    |     aFcnTruthTableAction_5();
    | else % Default
    |     aFcnTruthTableAction_5();
    | end
    | 
    | function aFcnTruthTableAction_1()
    | 
    | % FastTwitch
    | 
    | poseType=13;
    | 
    | function aFcnTruthTableAction_2()
    | 
    | % SlowTwitch
    | 
    | poseType=14;
    | 
    | function aFcnTruthTableAction_3()
    | 
    | % FastNoTwitch
    | 
    | poseType=23;
    | 
    | function aFcnTruthTableAction_4()
    | 
    | % SlowNoTwitch
    | 
    | poseType=24;
    | 
    | function aFcnTruthTableAction_5()
    | 
    | % normal
    | 
    | poseType=27;
  function newBmls =insertQueueLow(bmls,myBML):
    | function newBmls =insertQueueLow(bmls,myBML)
    |     full=1;
    |     t=encStr2Arr(' ');
    |     newBmls=[t t t t t];
    |     for i = 1:5
    |         if (isequal(bmls(:,i),t))
    |             %add to end of the queue where its empty
    |             bmls(:,i)=myBML;
    |             full=0;
    |             break
    |         end
    |     end
    |     if(full~=0)
    |             %if queue full, shift all elements to left which removes the first one, then add to end
    |             bmls(:,1)= bmls(:,2);
    |             bmls(:,2)= bmls(:,3);
    |             bmls(:,3)= bmls(:,4);
    |             bmls(:,5)=myBML;
    |     end
    |     newBmls=bmls;
  function newBmls =insertQueue(bmls,myBML):
    | function newBmls =insertQueue(bmls,myBML)
    |     full=1;
    |     t=encStr2Arr(' ');
    |     newBmls=[t t t t t];
    |     for i = 1:5
    |         if (isequal(bmls(:,i),t))
    |             %add to end of the queue where its empty
    |             bmls(:,i)=myBML;
    |             full=0;
    |             break
    |         end
    |     end
    |     if(full~=0)
    |             %if queue full, shift all elements to left which removes the first one, then add to end
    |             bmls(:,1)= bmls(:,2);
    |             bmls(:,2)= bmls(:,3);
    |             bmls(:,3)= bmls(:,4);
    |             bmls(:,5)=myBML;
    |     end
    |     newBmls=bmls;

== matlab function Expriment_All2/moveFWTable ==
  data: z input; y output
function y = fcn(z)

aVarTruthTableCondition_1 = false;
aVarTruthTableCondition_2 = false;
aVarTruthTableCondition_3 = false;
aVarTruthTableCondition_4 = false;


% too far

aVarTruthTableCondition_1 = logical(z >= 220);

% too close

aVarTruthTableCondition_2 = logical(z < 150 && z~=0);

% properSpace

aVarTruthTableCondition_3 = logical(z>=150 && z<220);

% no value

aVarTruthTableCondition_4 = logical(z==0);

if (aVarTruthTableCondition_1)
    aFcnTruthTableAction_1();
elseif (aVarTruthTableCondition_2)
    aFcnTruthTableAction_2();
elseif (aVarTruthTableCondition_3)
    aFcnTruthTableAction_3();
elseif (aVarTruthTableCondition_4)
    aFcnTruthTableAction_4();
else % Default
    aFcnTruthTableAction_4();
end

function aFcnTruthTableAction_1()

% too far

y = 2;

function aFcnTruthTableAction_2()

% too close

y = 1;

function aFcnTruthTableAction_3()

% properSpace

y = 0;

function aFcnTruthTableAction_4()

% no value

y = 3;

== matlab function Expriment_All2/gazeTable ==
  data: x input; y output
function y = fcn(x)

aVarTruthTableCondition_1 = false;
aVarTruthTableCondition_2 = false;


% moved left

aVarTruthTableCondition_1 = logical(x > 50);

% moved right

aVarTruthTableCondition_2 = logical(x < -50);

if (aVarTruthTableCondition_1)
    aFcnTruthTableAction_1();
elseif (aVarTruthTableCondition_2)
    aFcnTruthTableAction_2();
else % Default
    aFcnTruthTableAction_3();
end

function aFcnTruthTableAction_1()

% moved left

y = 1;

function aFcnTruthTableAction_2()

% moved right

y = 2;

function aFcnTruthTableAction_3()

% proper place

y = 0;
